simulink library "wind_gust_lib"  (R2024b)
settings: Solver=ode45  StartTime=0.0  StopTime=10.0  RelTol=1e-3
undefined symbols (not defined in the file): a, b, Mq, Mw, Swg, Vto, Zw
libraries: simulink x1
settings Model: ModifiedByFormat=The MathWorks Inc.  Creator=The MathWorks, Inc.  LastModifiedBy=The MathWorks Inc.
settings SolverCC: DateTimeAtSimulationTimeZero=[]  AlgebraicLoopSolver=TrustRegion
settings DataIOCC: LimitDataPoints=on  SaveFormat=Array  SignalLoggingSaveFormat=ModelDataLogs  ReturnWorkspaceOutputs=off
settings OptimizationCC: BlockReduction=off  BooleanDataType=off  ExpressionDepthLimit=2147483647  LifeSpan=inf
settings DebuggingCC: SaveWithParameterizedLinksMsg=none  UnderspecifiedInitializationDetection=Classic  MergeDetectMultiDrivingBlocksExec=none  SignalResolutionControl=TryResolveAllWithWarning  FcnCallInpInsideContextMsg=warning  UnconnectedInputMsg=warning  UnconnectedOutputMsg=warning  UnconnectedLineMsg=warning  StateNameClashWarn=warning  SFUnexpectedBacktrackingDiag=warning  SFNoUnconditionalDefaultTransitionDiag=warning  SFExecutionAtInitializationDiag=none  ArithmeticOperatorsInVariantConditions=warning
settings HardwareCC: ProdBitPerPointer=32  ProdBitPerSizeT=32  ProdBitPerPtrDiffT=32  ProdLargestAtomicFloat=None  ProdIntDivRoundTo=Undefined  ProdEndianess=Unspecified  ProdWordSize=32  ProdHWDeviceType=32-bit Generic  TargetUnknown=on
settings ModelReferenceCC: EnableRefExpFcnMdlSchedulingChecks=on  PropagateSignalLabelsOutOfModel=off
settings SFSimCC: SimUseLocalCustomCode=off  CustomCodeUndefinedFunction=UseInterfaceOnly
settings RTWCC: RTWUseLocalCustomCode=off  GPUComputeCapability=3.5
settings CodeAppCC: StateflowObjectComments=on
settings GRTTargetCC: TargetLangStandard=C89/C90 (ANSI)  CombineOutputUpdateFcns=off  GRTInterface=on
settings ConfigComp: CovMetricSettings=dw  CovSaveCumulativeToWorkspaceVar=on  CovSaveSingleToWorkspaceVar=on  CovExternalEMLEnable=off

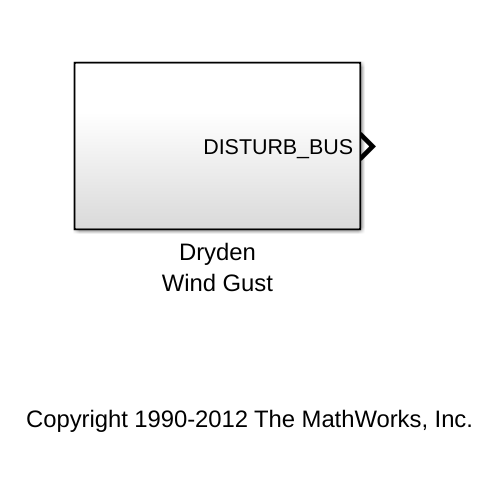
[thumbnail: Simulink's stored preview of the top-level diagram]
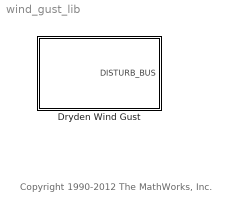
== system wind_gust_lib ==
  note: Copyright 1990-2012 The MathWorks, Inc.
  Dryden Wind Gust : Subsystem

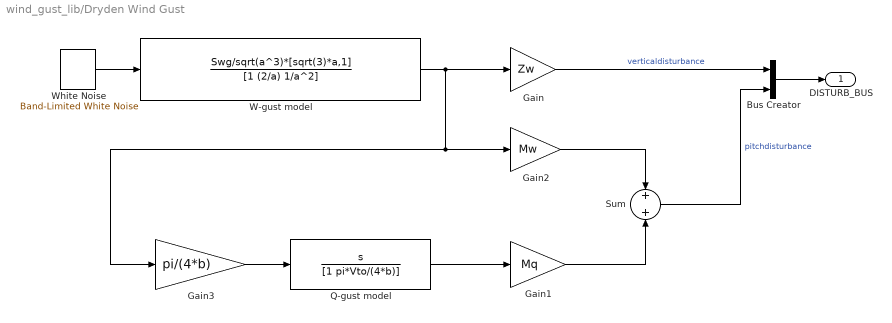
== system wind_gust_lib/Dryden Wind Gust ==
  Bus Creator : BusCreator  Inputs='verticaldisturbance','pitchdisturbance'  OutDataTypeStr=Bus: DISTURB_BUS
  Gain : Gain  Gain=Zw  SaturateOnIntegerOverflow=on  OutDataTypeStr=Inherit: Same as input  ParamDataTypeStr=Inherit: Same as input
  Gain1 : Gain  Gain=Mq  SaturateOnIntegerOverflow=on  OutDataTypeStr=Inherit: Same as input  ParamDataTypeStr=Inherit: Same as input
  Gain2 : Gain  Gain=Mw  SaturateOnIntegerOverflow=on  OutDataTypeStr=Inherit: Same as input  ParamDataTypeStr=Inherit: Same as input
  Gain3 : Gain  Gain=pi/(4*b)  SaturateOnIntegerOverflow=on  OutDataTypeStr=Inherit: Same as input  ParamDataTypeStr=Inherit: Same as input
  Q-gust model : TransferFcn  Numerator=[1 0]  Denominator=[1 pi*Vto/(4*b)]
  Sum : Sum  InputSameDT=on  SaturateOnIntegerOverflow=on  OutDataTypeStr=Inherit: Same as first input
  W-gust model : TransferFcn  Numerator=Swg/sqrt(a^3)*[sqrt(3)*a,1]  Denominator=[1 (2/a) 1/a^2]
  White Noise : simulink/Sources/Band-Limited White Noise  Cov=10  Ts=0.01  seed=23341
  DISTURB_BUS : Outport  OutDataTypeStr=Bus: DISTURB_BUS
  wires:
  Bus Creator/1 -> DISTURB_BUS/1
  Gain/1 -> Bus Creator/1  "verticaldisturbance"
  White Noise/1 -> W-gust model/1
  Gain3/1 -> Q-gust model/1
  Sum/1 -> Bus Creator/2  "pitchdisturbance"
  Gain2/1 -> Sum/1
  Gain1/1 -> Sum/2
  Q-gust model/1 -> Gain1/1
  W-gust model/1 -> Gain/1, Gain2/1, Gain3/1
